simulink model "na_dendrite_soma"  (R2020b)
settings: Solver=VariableStepAuto  StartTime=0  StopTime=t_end_ms  MaxStep=t_step  RelTol=1e-3
values from neighbouring files (symbols this model uses):
  gain = gain_arr(k)    [run_parallel_sims.m]    (also in run_single_sim.m = 3)
  loc = loc_arr(j)    [run_parallel_sims.m]    (also in run_single_sim.m = 2)
  peak = peak_arr(i)    [run_parallel_sims.m]    (also in run_single_sim.m = 1.95)
  pulse_height = pulse_height_arr(m)    [run_parallel_sims.m]    (also in run_single_sim.m = 1.5)
  pulse_width_ms = 1    [run_parallel_sims.m]    (also in run_single_sim.m)
  sensitivity = 0.35    [run_single_sim.m]
  soma_threshold = 0.23    [run_single_sim.m]
libraries: simulink x1
settings Model: SimulationMode=accelerator  Creator=Peter  LastModifiedBy=prshe

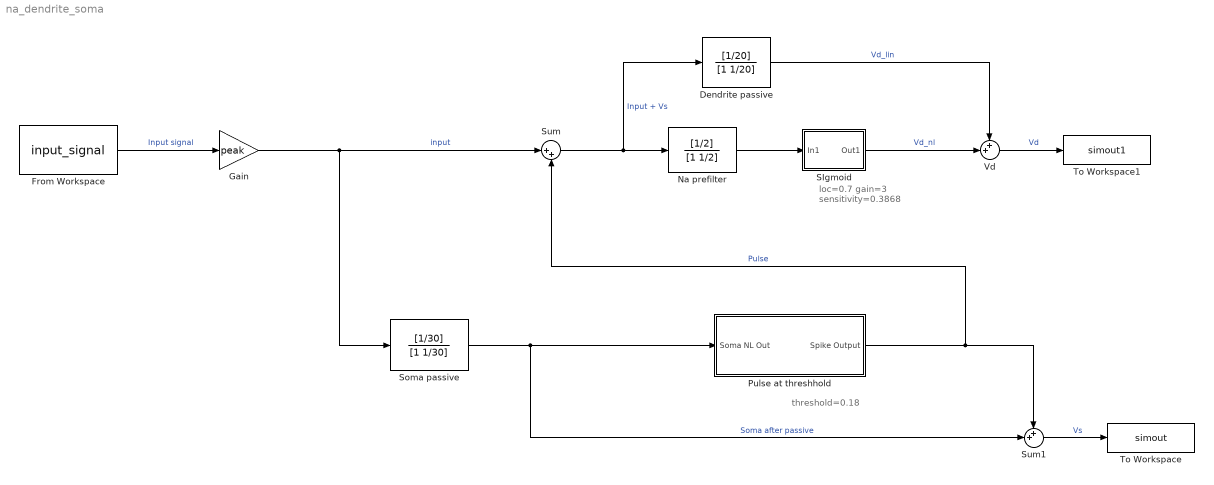
== system na_dendrite_soma ==
  note: threshold=0.18
  note: loc=0.7
      | gain=3
      | sensitivity=0.3868
  Dendrite passive : TransferFcn  Numerator=[1/20]  Denominator=[1 1/20]
  From Workspace : FromWorkspace  VariableName=input_signal
  Gain : Gain  Gain=peak
  Na prefilter : TransferFcn  Numerator=[1/2]  Denominator=[1 1/2]
  Pulse at threshhold : Subsystem
  SIgmoid : Subsystem  mask{Loc=loc, Gain=gain, Sensitivity=sensitivity}
      mask TypeOptions Loc: loc/Value
      mask TypeOptions Gain: Gain1/Gain
      mask TypeOptions Sensitivity: sensitivity/Value
  Soma passive : TransferFcn  Numerator=[1/30]  Denominator=[1 1/30]
  Sum : Sum  Inputs=|++
  Sum1 : Sum  Inputs=++|
  To Workspace : ToWorkspace  VariableName=simout  SaveFormat=Timeseries  SampleTime=-1
  To Workspace1 : ToWorkspace  VariableName=simout1  SaveFormat=Timeseries  SampleTime=-1
  Vd : Sum  Inputs=++|
  wires:
  Na prefilter/1 -> SIgmoid/1(In1)
  SIgmoid/1(Out1) -> Vd/2  "Vd_nl"
  Dendrite passive/1 -> Vd/1  "Vd_lin"
  Vd/1 -> To Workspace1/1  "Vd"
  Sum/1 -> Dendrite passive/1, Na prefilter/1  "Input + Vs"
  Soma passive/1 -> Pulse at threshhold/1(Soma NL Out), Sum1/2  "Soma after passive"
  Sum1/1 -> To Workspace/1  "Vs"
  Pulse at threshhold/1(Spike Output) -> Sum1/1, Sum/2  "Pulse"
  Gain/1 -> Soma passive/1, Sum/1  "input"
  From Workspace/1 -> Gain/1  "Input signal"

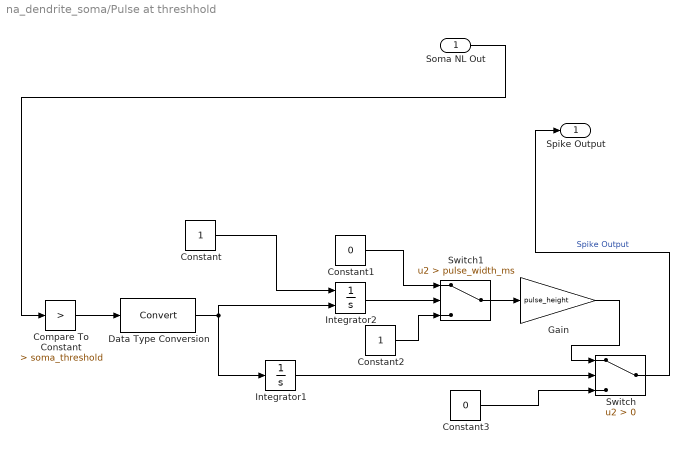
== system na_dendrite_soma/Pulse at threshhold ==
  Soma NL Out : Inport
  Compare To Constant : simulink/Logic and Bit Operations/Compare To Constant  relop=>  const=soma_threshold  OutDataTypeStr=boolean
  Constant : Constant
  Constant1 : Constant  Value=0
  Constant2 : Constant
  Constant3 : Constant  Value=0
  Data Type Conversion : DataTypeConversion  RndMeth=Round
  Gain : Gain  Gain=pulse_height
  Integrator1 : Integrator
  Integrator2 : Integrator  ExternalReset=rising
  Switch : Switch  Criteria=u2 > Threshold
  Switch1 : Switch  Criteria=u2 > Threshold  Threshold=pulse_width_ms
  Spike Output : Outport
  wires:
  Integrator1/1 -> Switch/2
  Compare To Constant/1 -> Data Type Conversion/1
  Data Type Conversion/1 -> Integrator1/1, Integrator2/2
  Soma NL Out/1 -> Compare To Constant/1
  Switch/1 -> Spike Output/1  "Spike Output"
  Constant/1 -> Integrator2/1
  Integrator2/1 -> Switch1/2
  Constant2/1 -> Switch1/3
  Constant1/1 -> Switch1/1
  Constant3/1 -> Switch/3
  Switch1/1 -> Gain/1
  Gain/1 -> Switch/1

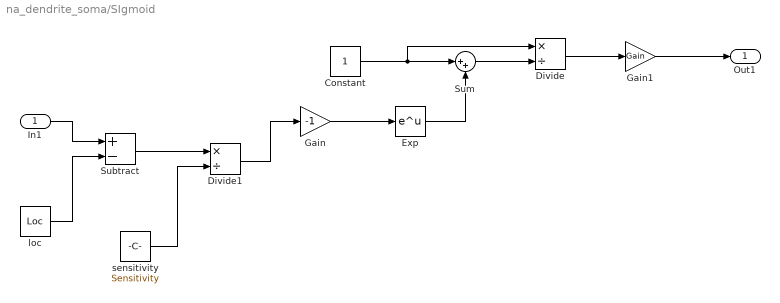
== system na_dendrite_soma/SIgmoid ==
  In1 : Inport
  Constant : Constant
  Divide : Product  Inputs=*/
  Divide1 : Product  Inputs=*/
  Exp : Math  SaturateOnIntegerOverflow=on
  Gain : Gain  Gain=-1
  Gain1 : Gain  Gain=Gain
  Subtract : Sum  Inputs=+-
  Sum : Sum  Inputs=|++
  loc : Constant  Value=Loc
  sensitivity : Constant  Value=Sensitivity
  Out1 : Outport
  wires:
  Gain/1 -> Exp/1
  Constant/1 -> Divide/1, Sum/1
  Exp/1 -> Sum/2
  Sum/1 -> Divide/2
  In1/1 -> Subtract/1
  loc/1 -> Subtract/2
  Subtract/1 -> Divide1/1
  sensitivity/1 -> Divide1/2
  Divide1/1 -> Gain/1
  Divide/1 -> Gain1/1
  Gain1/1 -> Out1/1
